simulink model "PropellerModel"  (R2022b)
settings: Solver=VariableStepAuto  StartTime=0.0  StopTime=500  RelTol=1e-3
libraries: mssSimulink x1
settings Model: PacingRate=10  Creator=Lenovo  LastModifiedBy=ADMIN
settings ModelReferenceCC: EnableRefExpFcnMdlSchedulingChecks=on

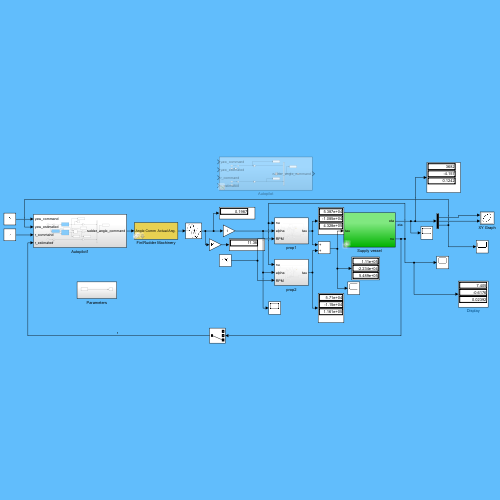
[thumbnail: Simulink's stored preview of the top-level diagram]
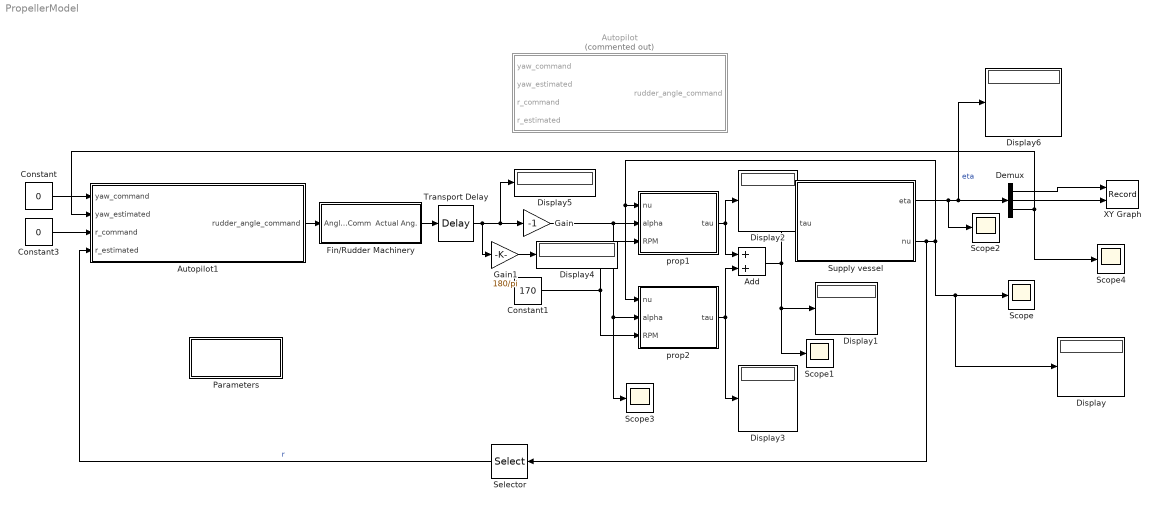
== system PropellerModel ==
  Add : Sum
  Autopilot : Subsystem  Commented=on
  Autopilot1 : Subsystem
  Constant : Constant  Value=0
  Constant1 : Constant  Value=170
  Constant3 : Constant  Value=0
  Demux : Demux  Outputs=3
  Display{,1..6} (7 alike) : Display
  Fin/Rudder Machinery : Subsystem  AncestorBlock=mssSimulink/Modelling/Control Surfaces/Fin//Rudder Machinery  mask(Rudder Machinery){Dmax=20, Dvmax=2*pi*1000/180, tc=.1}
      mask prompts: Dmax "Max. Rudder Angle (rad):"; Dvmax "Max. Rudder Rate (rad/sec.):"; tc "Time constant (sec):"
      mask help:
      | Model of van Amerongen for rudder machiery
      | Copyright (C) 2005 NTNU
      | Author: Tristan Perez
      settings: LibrarySourceBlock=mssSimulink/Modelling/Control Surfaces/Fin//Rudder Machinery
      mask Help: Rudder machinery model of Van Amerongen accounting for saturation and rate limit.
  Gain : Gain  Gain=-1
  Gain1 : Gain  Gain=180/pi
  Parameters : Subsystem
  Scope{,1..4} (5 alike) : Scope
  Selector : Selector  InputPortWidth=3  IndexOptions=Index vector (dialog)  Indices=[3]  OutputSizes=1
  Supply vessel : Subsystem  AncestorBlock=mssSimulink/Marine craft models/Supply vessel
      settings: LibrarySourceBlock=mssSimulink/Marine craft models/Supply vessel
  Transport Delay : TransportDelay  DelayTime=3
  XY Graph : Record  RecordToWorkspace=on  FileSettingsInternal="{\"entries\":[{\"content\":{\"excelSettings\":{\"content\":{},\"type\":\"Streamout.ExcelSettings\"}},\"type\":\"Streamout.FileSettingStorage\",\"uuid\":\"4c8f667d-2ec8-40bb-a75c-241daf6926ec\"}],\"packageUris\":[\"http://schema.mathworks.com/mf0/streamout_blocks/R2020a\"],\"version\":\"1.0\"}"  Layout=[1 1]  SignalsInternal="{\"entries\":[{\"content\":{\"signals\":[{\"content\":{\"blockPath\":[\"PropellerModel/XY Graph\"],\"channel\":[],\"dimensions\":[1],\"domain\":\"PropellerModel/XY Graph\",\"lineColor\":\"#a2142f\",\"plots\":[1],\"port\":1,\"sid\":[\"\"],\"signalID\":30923,\"signalName\":\"Demux:1\"},\"type\":\"RecordBlkView.Signal\",\"uuid\":\"623a59a8-df64-41e8-a8fb-f785ae9d3377\"},{\"content\":{\"blockPath\":[\"PropellerModel/XY Graph\"],\"channel\":[],\"dimensions\":[1],\"domain\":\"PropellerModel/XY Graph\",\"lineColor\":\"#139fff\",\"plots\":[1],\"port\":2,\"sid\":[\"\"],\"signalID\":30927,\"signalName\":\"Demux:2\"},\"type\":\"RecordBlkView.Signal\",\"uuid\":\"a734874c-224f-4494-ab74-00e3b52a102c\"}]},\"type\":\"RecordBlkView.InputSignals\",\"uuid\":\"024bf6ff-c6de-4f18-8bef-f27dde48d678\"}],\"packageUris\":[\"http://schema.mathworks.com/mf0/streamout_blocks/R2020a\"],\"version\":\"1.0\"}"  VisualizationBindings="{\"xyplotplugin\":{\"info\":[{\"series\":[{\"bindingParametersList\":[{\"parameter\":\"X-Axis\",\"signalID\":30923,\"signalName\":\"Demux:1\"},{\"parameter\":\"Y-Axis\",\"signalID\":30927,\"signalName\":\"Demux:2\"}],\"seriesID\":59875}],\"subplotID\":1}]}}"  CompatibilityTag=XY
  prop1 : Subsystem
  prop2 : Subsystem
  wires:
  Supply vessel/2(nu) -> Selector/1, Display/1, Scope/1, prop2/1(nu), prop1/1(nu)
  Autopilot1/1(rudder_angle_command) -> Fin/Rudder Machinery/1(Angle Comm)
  Supply vessel/1(eta) -> Scope2/1, Display6/1, Demux/1  "eta"
  Demux/1 -> XY Graph/1
  Demux/2 -> XY Graph/2
  Constant1/1 -> prop2/3(RPM), prop1/3(RPM)
  prop1/1(tau) -> Add/1, Display2/1
  prop2/1(tau) -> Add/2, Display3/1
  Add/1 -> Scope1/1, Display1/1, Supply vessel/1(tau)
  Fin/Rudder Machinery/1("Actual Ang. ") -> Transport Delay/1
  Constant/1 -> Autopilot1/1(yaw_command)
  Constant3/1 -> Autopilot1/3(r_command)
  Demux/3 -> Scope4/1, Autopilot1/2(yaw_estimated)
  Selector/1 -> Autopilot1/4(r_estimated)  "r"
  Gain/1 -> prop2/2(alpha), Scope3/1, prop1/2(alpha)
  Gain1/1 -> Display4/1
  Transport Delay/1 -> Gain1/1, Display5/1, Gain/1

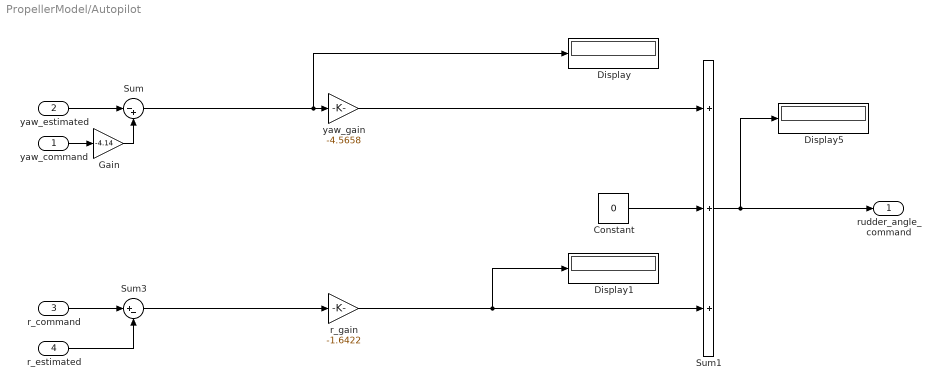
== system PropellerModel/Autopilot ==
  yaw_command : Inport
  yaw_estimated : Inport  Port=2
  r_command : Inport  Port=3
  r_estimated : Inport  Port=4
  Constant : Constant  Value=0
  Display : Display
  Display1 : Display
  Display5 : Display
  Gain : Gain  Gain=-4.14
  Sum : Sum  Inputs=|-+
  Sum1 : Sum  Inputs=+++  InputSameDT=on  SaturateOnIntegerOverflow=on  OutDataTypeStr=Inherit: Same as first input
  Sum3 : Sum  Inputs=|+-  InputSameDT=on  SaturateOnIntegerOverflow=on  OutDataTypeStr=Inherit: Same as first input
  r_gain : Gain  Gain=-1.6422
  yaw_gain : Gain  Gain=-4.5658
  rudder_angle_command : Outport
  wires:
  r_gain/1 -> Display1/1, Sum1/3
  Sum3/1 -> r_gain/1
  Sum1/1 -> Display5/1, rudder_angle_command/1
  r_estimated/1 -> Sum3/2
  r_command/1 -> Sum3/1
  yaw_estimated/1 -> Sum/1
  Sum/1 -> Display/1, yaw_gain/1
  yaw_gain/1 -> Sum1/1
  Constant/1 -> Sum1/2
  yaw_command/1 -> Gain/1
  Gain/1 -> Sum/2

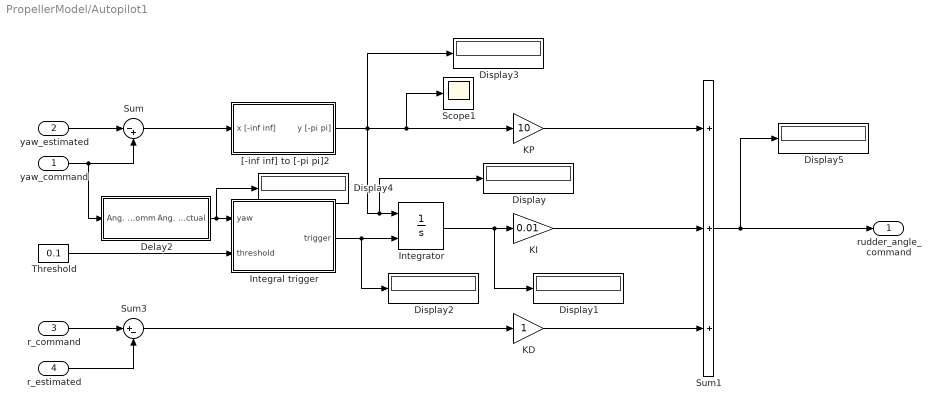
== system PropellerModel/Autopilot1 ==
  yaw_command : Inport
  yaw_estimated : Inport  Port=2
  r_command : Inport  Port=3
  r_estimated : Inport  Port=4
  Delay2 : Subsystem
  Display{,1..5} (6 alike) : Display
  Integral trigger : MATLAB Function  TreatAsAtomicUnit=on
  Integrator : Integrator  ExternalReset=level hold  LimitOutput=on  UpperSaturationLimit=deg2rad(20)  LowerSaturationLimit=deg2rad(-20)
  KD : Gain
  KI : Gain  Gain=0.01
  KP : Gain  Gain=10
  Scope1 : Scope
  Sum : Sum  Inputs=|-+
  Sum1 : Sum  Inputs=+++  InputSameDT=on  SaturateOnIntegerOverflow=on  OutDataTypeStr=Inherit: Same as first input
  Sum3 : Sum  Inputs=|+-  InputSameDT=on  SaturateOnIntegerOverflow=on  OutDataTypeStr=Inherit: Same as first input
  Threshold : Constant  Value=0.1
  "[-inf inf] to [-pi pi]2" : Subsystem  AncestorBlock=mssSimulink/Utilities/Math Operations/[-inf inf] to [-pi pi]  mask([-inf inf] to [-pi pi]){}
      mask help: Converts an angle in rad to (-pi pi)
      settings: LibrarySourceBlock=mssSimulink/Utilities/Math Operations/[-inf inf] to [-pi pi]
  rudder_angle_command : Outport
  wires:
  Integrator/1 -> Display1/1, KI/1
  KD/1 -> Sum1/3
  Sum/1 -> "[-inf inf] to [-pi pi]2"/1(x [-inf inf])
  Sum3/1 -> KD/1
  "[-inf inf] to [-pi pi]2"/1(y [-pi pi]) -> Scope1/1, KP/1, Display3/1, Display/1, Integrator/1
  KI/1 -> Sum1/2
  Sum1/1 -> Display5/1, rudder_angle_command/1
  r_estimated/1 -> Sum3/2
  r_command/1 -> Sum3/1
  yaw_estimated/1 -> Sum/1
  KP/1 -> Sum1/1
  Integral trigger/1(trigger) -> Display2/1, Integrator/2
  Threshold/1 -> Integral trigger/2(threshold)
  yaw_command/1 -> Sum/2, Delay2/1(Ang. Comm)
  Delay2/1(Ang. Actual) -> Display4/1, Integral trigger/1(yaw)

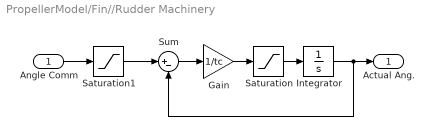
== system PropellerModel/Fin//Rudder Machinery ==
  Angle Comm : Inport
  Gain : Gain  Gain=1/tc  SaturateOnIntegerOverflow=on  OutDataTypeStr=Inherit: Same as input  ParamDataTypeStr=Inherit: Same as input
  Integrator : Integrator
  Saturation : Saturate  UpperLimit=deg2rad(3)  LowerLimit=-deg2rad(3)
  Saturation1 : Saturate  UpperLimit=deg2rad(Dmax)  LowerLimit=deg2rad(-Dmax)
  Sum : Sum  Inputs=|+-  InputSameDT=on  SaturateOnIntegerOverflow=on  OutDataTypeStr=Inherit: Same as first input
  "Actual Ang. " : Outport  VectorParamsAs1DForOutWhenUnconnected=off
  wires:
  Gain/1 -> Saturation/1
  Sum/1 -> Gain/1
  Integrator/1 -> Sum/2, "Actual Ang. "/1
  Saturation1/1 -> Sum/1
  Saturation/1 -> Integrator/1
  Angle Comm/1 -> Saturation1/1

== system PropellerModel/Parameters ==
  Mass : Constant  Value=357.0*1014
  tag scope: Mass=global
  wires:
  Mass/1 -> [Mass]

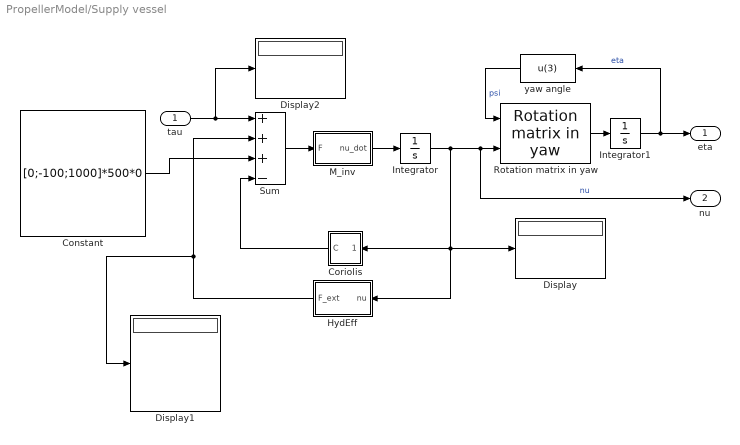
== system PropellerModel/Supply vessel ==
  tau : Inport
  Constant : Constant  Value=[0;-100;1000]*500*0
  Coriolis : Subsystem
  Display : Display
  Display1 : Display
  Display2 : Display
  HydEff : Subsystem
  Integrator : Integrator  InitialCondition=[0 1 0]
  Integrator1 : Integrator
  M_inv : Subsystem
  "Rotation matrix in yaw " : mssSimulink/Modelling/Kinematics/Rotation matrix in yaw 
  Sum : Sum  Inputs=+++-  InputSameDT=on  SaturateOnIntegerOverflow=on  OutDataTypeStr=Inherit: Same as first input
  yaw angle : Fcn  Expr=u(3)
  eta : Outport  InitialOutput=0  VectorParamsAs1DForOutWhenUnconnected=off
  nu : Outport  Port=2  InitialOutput=0  VectorParamsAs1DForOutWhenUnconnected=off
  wires:
  Sum/1 -> M_inv/1(F)
  M_inv/1(nu_dot) -> Integrator/1
  tau/1 -> Display2/1, Sum/1
  "Rotation matrix in yaw "/1 -> Integrator1/1
  yaw angle/1 -> "Rotation matrix in yaw "/1  "psi"
  Integrator/1 -> Display/1, HydEff/1(nu), Coriolis/1(nu), "Rotation matrix in yaw "/2, nu/1  "nu"
  Integrator1/1 -> yaw angle/1, eta/1  "eta"
  HydEff/1(F_ext) -> Display1/1, Sum/2
  Coriolis/1(C) -> Sum/4
  Constant/1 -> Sum/3

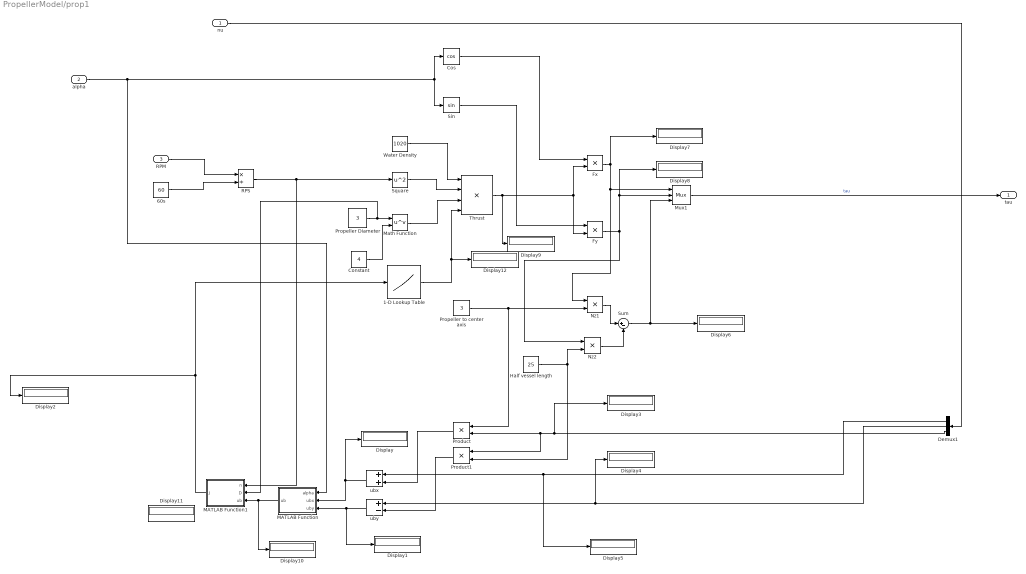
== system PropellerModel/prop1 ==
  nu : Inport
  alpha : Inport  Port=2
  RPM : Inport  Port=3
  1-D Lookup Table : Lookup_n-D  NumberOfTableDimensions=1  BreakpointsForDimension1=[0:0.05:1.05]  Table=-0.3*[0:0.05:1.05]+0.35  InternalRulePriority=Speed  RndMeth=Simplest
  60s : Constant  Value=60
  Constant : Constant  Value=4
  Cos : Trigonometry  Operator=cos
  Demux1 : Demux  Outputs=3
  Display{,1..12} (13 alike) : Display
  Fx : Product
  Fy : Product
  Half vessel length : Constant  Value=25
  MATLAB Function : MATLAB Function  TreatAsAtomicUnit=on
  MATLAB Function1 : MATLAB Function  TreatAsAtomicUnit=on
  Math Function : Math  Operator=pow
  Mux1 : Mux  Inputs=3
  Nz1 : Product
  Nz2 : Product
  Product : Product
  Product1 : Product
  "Propeller Diameter " : Constant  Value=3
  Propeller to center axis : Constant  Value=3
  RPS : Product  Inputs=*/  RndMeth=Zero  SaturateOnIntegerOverflow=on
  Sin : Trigonometry
  Square : Math  Operator=square
  Sum : Sum  Inputs=|+-
  Thrust : Product  Inputs=4
  Water Density : Constant  Value=1020
  ubx : Sum
  uby : Sum  Inputs=+-
  tau : Outport
  wires:
  nu/1 -> Demux1/1
  Nz2/1 -> Sum/2
  alpha/1 -> Cos/1, Sin/1, MATLAB Function/1(alpha)
  RPS/1 -> Square/1, MATLAB Function1/1(n)
  Half vessel length/1 -> Product1/2, Nz2/2
  Fy/1 -> Display8/1, Mux1/2, Nz2/1
  Water Density/1 -> Thrust/1
  uby/1 -> MATLAB Function/3(uby), Display1/1
  Propeller to center axis/1 -> Product/1, Nz1/2
  Thrust/1 -> Display9/1, Fy/2, Fx/2
  Fx/1 -> Mux1/1, Nz1/1, Display7/1
  Square/1 -> Thrust/2
  Demux1/2 -> Display4/1, uby/1
  MATLAB Function/1(ub) -> Display10/1, MATLAB Function1/3(ub)
  60s/1 -> RPS/2
  Cos/1 -> Fx/1
  Demux1/1 -> Display5/1, ubx/1
  Sum/1 -> Display6/1, Mux1/3
  ubx/1 -> MATLAB Function/2(ubx), Display/1
  Nz1/1 -> Sum/1
  MATLAB Function1/1(J) -> 1-D Lookup Table/1, Display2/1
  1-D Lookup Table/1 -> Thrust/4, Display12/1
  Mux1/1 -> tau/1  "tau"
  RPM/1 -> RPS/1
  Demux1/3 -> Display3/1, Product1/1, Product/2
  Product/1 -> ubx/2
  Product1/1 -> uby/2
  Sin/1 -> Fy/1
  "Propeller Diameter "/1 -> Math Function/1, MATLAB Function1/2(D)
  Constant/1 -> Math Function/2
  Math Function/1 -> Thrust/3

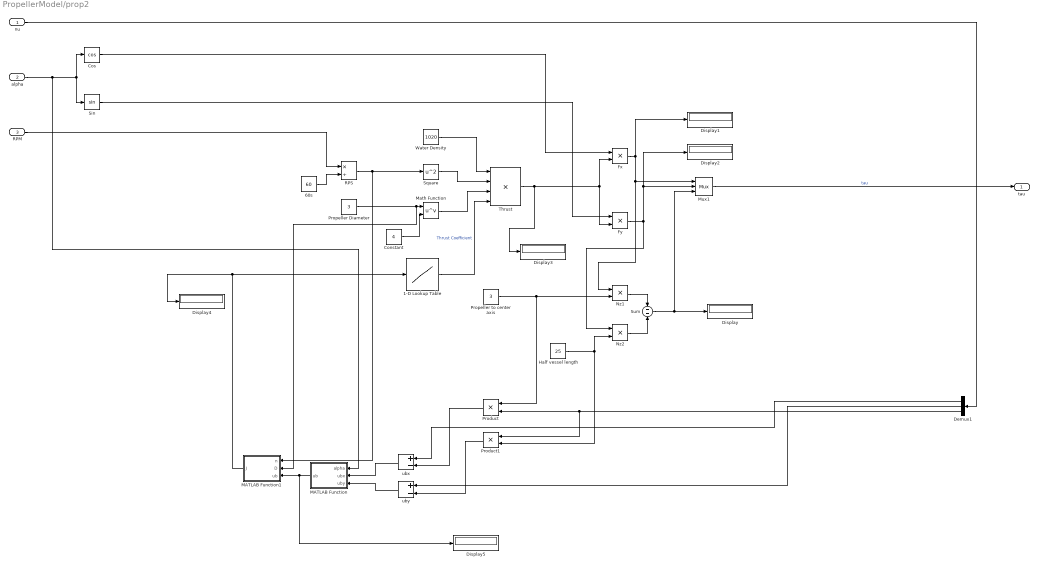
== system PropellerModel/prop2 ==
  nu : Inport
  alpha : Inport  Port=2
  RPM : Inport  Port=3
  1-D Lookup Table : Lookup_n-D  NumberOfTableDimensions=1  BreakpointsForDimension1=[0:0.05:1.05]  Table=-0.3*[0:0.05:1.05]+0.35  InternalRulePriority=Speed  RndMeth=Simplest
  60s : Constant  Value=60
  Constant : Constant  Value=4
  Cos : Trigonometry  Operator=cos
  Demux1 : Demux  Outputs=3
  Display{,1..5} (6 alike) : Display
  Fx : Product
  Fy : Product
  Half vessel length : Constant  Value=25
  MATLAB Function : MATLAB Function  TreatAsAtomicUnit=on
  MATLAB Function1 : MATLAB Function  TreatAsAtomicUnit=on
  Math Function : Math  Operator=pow
  Mux1 : Mux  Inputs=3
  Nz1 : Product
  Nz2 : Product
  Product : Product
  Product1 : Product
  Propeller Diameter : Constant  Value=3
  Propeller to center axis : Constant  Value=3
  RPS : Product  Inputs=*/  RndMeth=Zero  SaturateOnIntegerOverflow=on
  Sin : Trigonometry
  Square : Math  Operator=square
  Sum : Sum  Inputs=--
  Thrust : Product  Inputs=4
  Water Density : Constant  Value=1020
  ubx : Sum  Inputs=+-
  uby : Sum  Inputs=+-
  tau : Outport
  wires:
  Product1/1 -> uby/2
  Product/1 -> ubx/2
  Demux1/3 -> Product1/1, Product/2
  RPM/1 -> RPS/1
  Mux1/1 -> tau/1  "tau"
  1-D Lookup Table/1 -> Thrust/4  "Thrust Coefficient"
  MATLAB Function1/1(J) -> Display4/1, 1-D Lookup Table/1
  Nz1/1 -> Sum/1
  Sum/1 -> Mux1/3, Display/1
  60s/1 -> RPS/2
  Demux1/2 -> uby/1
  Square/1 -> Thrust/2
  Propeller Diameter/1 -> MATLAB Function1/2(D), Math Function/1
  Fx/1 -> Nz1/1, Mux1/1, Display1/1
  Thrust/1 -> Display3/1, Fx/2, Fy/2
  Propeller to center axis/1 -> Nz1/2, Product/1
  Water Density/1 -> Thrust/1
  Fy/1 -> Nz2/1, Display2/1, Mux1/2
  Half vessel length/1 -> Nz2/2, Product1/2
  RPS/1 -> Square/1, MATLAB Function1/1(n)
  alpha/1 -> MATLAB Function/1(alpha), Sin/1, Cos/1
  Nz2/1 -> Sum/2
  nu/1 -> Demux1/1
  Cos/1 -> Fx/1
  Sin/1 -> Fy/1
  Math Function/1 -> Thrust/3
  Constant/1 -> Math Function/2
  Demux1/1 -> ubx/1
  ubx/1 -> MATLAB Function/2(ubx)
  uby/1 -> MATLAB Function/3(uby)
  MATLAB Function/1(ub) -> Display5/1, MATLAB Function1/3(ub)

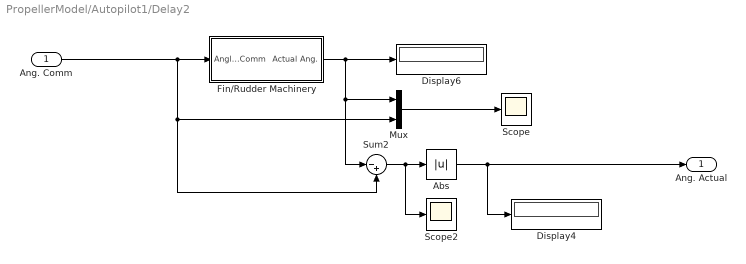
== system PropellerModel/Autopilot1/Delay2 ==
  Ang. Comm : Inport
  Abs : Abs  SaturateOnIntegerOverflow=off
  Display4 : Display
  Display6 : Display
  Fin/Rudder Machinery : Subsystem  AncestorBlock=mssSimulink/Modelling/Control Surfaces/Fin//Rudder Machinery  mask(Rudder Machinery){Dmax=20, Dvmax=0.05, tc=.005}
      mask prompts: Dmax "Max. Rudder Angle (rad):"; Dvmax "Max. Rudder Rate (rad/sec.):"; tc "Time constant (sec):"
      mask help:
      | Model of van Amerongen for rudder machiery
      | Copyright (C) 2005 NTNU
      | Author: Tristan Perez
      settings: LibrarySourceBlock=mssSimulink/Modelling/Control Surfaces/Fin//Rudder Machinery
      mask Help: Rudder machinery model of Van Amerongen accounting for saturation and rate limit.
  Mux : Mux  Inputs=2
  Scope : Scope
  Scope2 : Scope
  Sum2 : Sum  Inputs=|-+
  Ang. Actual : Outport
  wires:
  Sum2/1 -> Scope2/1, Abs/1
  Ang. Comm/1 -> Fin/Rudder Machinery/1(Angle Comm), Sum2/2, Mux/2
  Fin/Rudder Machinery/1("Actual Ang. ") -> Sum2/1, Mux/1, Display6/1
  Abs/1 -> Ang. Actual/1, Display4/1
  Mux/1 -> Scope/1

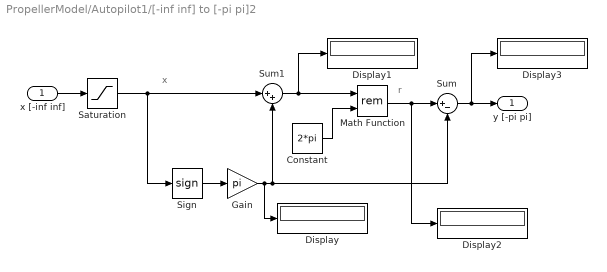
== system PropellerModel/Autopilot1/[-inf inf] to [-pi pi]2 ==
  note: x
  note: r
  x [-inf inf] : Inport
  Constant : Constant  Value=2*pi
  Display{,1..3} (4 alike) : Display
  Gain : Gain  Gain=pi  SaturateOnIntegerOverflow=on  OutDataTypeStr=Inherit: Same as input  ParamDataTypeStr=Inherit: Same as input
  Math Function : Math  Operator=rem  SignedPower=on
  Saturation : Saturate  UpperLimit=1e10  LowerLimit=-1e10
  Sign : Signum
  Sum : Sum  Inputs=|+-  SaturateOnIntegerOverflow=on
  Sum1 : Sum  Inputs=|++  SaturateOnIntegerOverflow=on
  y [-pi pi] : Outport  VectorParamsAs1DForOutWhenUnconnected=off
  wires:
  x [-inf inf]/1 -> Saturation/1
  Sign/1 -> Gain/1
  Gain/1 -> Display/1, Sum/2, Sum1/2
  Sum1/1 -> Display1/1, Math Function/1
  Constant/1 -> Math Function/2
  Sum/1 -> Display3/1, y [-pi pi]/1
  Saturation/1 -> Sum1/1, Sign/1
  Math Function/1 -> Display2/1, Sum/1

== system PropellerModel/Supply vessel/Coriolis ==
  nu : Inport
  Demux : Demux  Outputs=3
  Display : Display
  MATLAB Function : MATLAB Function  TreatAsAtomicUnit=on
  Mux : Mux  Inputs=3
  C : Outport
  wires:
  nu/1 -> Display/1, Demux/1
  MATLAB Function/2(C2) -> Mux/2
  MATLAB Function/3(C3) -> Mux/3
  MATLAB Function/1(C1) -> Mux/1
  Mux/1 -> C/1
  Demux/1 -> MATLAB Function/1(u)
  Demux/2 -> MATLAB Function/2(v)
  Demux/3 -> MATLAB Function/3(r)

== system PropellerModel/Supply vessel/HydEff ==
  nu : Inport
  Bus Creator : BusCreator  Inputs=3
  Demux : Demux  Outputs=3
  MATLAB Function : MATLAB Function  TreatAsAtomicUnit=on
  F_ext : Outport
  wires:
  [Mass] -> MATLAB Function/1(mass)
  MATLAB Function/1(Xh) -> Bus Creator/1
  Bus Creator/1 -> F_ext/1
  MATLAB Function/2(Yh) -> Bus Creator/2
  MATLAB Function/3(Nh) -> Bus Creator/3
  nu/1 -> Demux/1
  Demux/1 -> MATLAB Function/2(u)
  Demux/2 -> MATLAB Function/3(v)
  Demux/3 -> MATLAB Function/4(r)

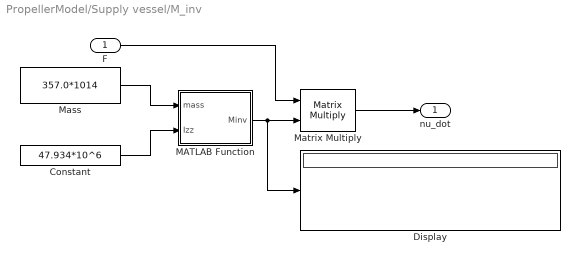
== system PropellerModel/Supply vessel/M_inv ==
  F : Inport
  Constant : Constant  Value=47.934*10^6
  Display : Display
  MATLAB Function : MATLAB Function  TreatAsAtomicUnit=on
  Mass : Constant  Value=357.0*1014
  Matrix Multiply : Product  Multiplication=Matrix(*)
  nu_dot : Outport
  wires:
  MATLAB Function/1(Minv) -> Display/1, Matrix Multiply/2
  Mass/1 -> MATLAB Function/1(mass)
  Constant/1 -> MATLAB Function/2(Izz)
  Matrix Multiply/1 -> nu_dot/1
  F/1 -> Matrix Multiply/1

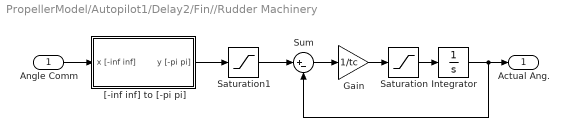
== system PropellerModel/Autopilot1/Delay2/Fin//Rudder Machinery ==
  Angle Comm : Inport
  Gain : Gain  Gain=1/tc  SaturateOnIntegerOverflow=on  OutDataTypeStr=Inherit: Same as input  ParamDataTypeStr=Inherit: Same as input
  Integrator : Integrator
  Saturation : Saturate  UpperLimit=Dvmax  LowerLimit=-Dvmax
  Saturation1 : Saturate  UpperLimit=Dmax  LowerLimit=-Dmax
  Sum : Sum  Inputs=|+-  InputSameDT=on  SaturateOnIntegerOverflow=on  OutDataTypeStr=Inherit: Same as first input
  "[-inf inf] to [-pi pi]" : Subsystem  AncestorBlock=mssSimulink/Utilities/Math Operations/[-inf inf] to [-pi pi]  mask([-inf inf] to [-pi pi]){}
      mask help: Converts an angle in rad to (-pi pi)
      settings: LibrarySourceBlock=mssSimulink/Utilities/Math Operations/[-inf inf] to [-pi pi]
  "Actual Ang. " : Outport  VectorParamsAs1DForOutWhenUnconnected=off
  wires:
  Gain/1 -> Saturation/1
  Sum/1 -> Gain/1
  Integrator/1 -> Sum/2, "Actual Ang. "/1
  Saturation1/1 -> Sum/1
  Saturation/1 -> Integrator/1
  Angle Comm/1 -> "[-inf inf] to [-pi pi]"/1(x [-inf inf])
  "[-inf inf] to [-pi pi]"/1(y [-pi pi]) -> Saturation1/1

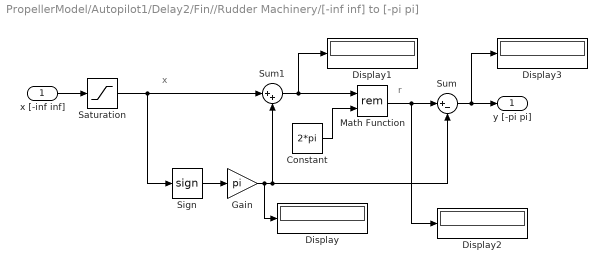
== system PropellerModel/Autopilot1/Delay2/Fin//Rudder Machinery/[-inf inf] to [-pi pi] ==
  note: x
  note: r
  x [-inf inf] : Inport
  Constant : Constant  Value=2*pi
  Display{,1..3} (4 alike) : Display
  Gain : Gain  Gain=pi  SaturateOnIntegerOverflow=on  OutDataTypeStr=Inherit: Same as input  ParamDataTypeStr=Inherit: Same as input
  Math Function : Math  Operator=rem  SignedPower=on
  Saturation : Saturate  UpperLimit=1e10  LowerLimit=-1e10
  Sign : Signum
  Sum : Sum  Inputs=|+-  SaturateOnIntegerOverflow=on
  Sum1 : Sum  Inputs=|++  SaturateOnIntegerOverflow=on
  y [-pi pi] : Outport  VectorParamsAs1DForOutWhenUnconnected=off
  wires:
  x [-inf inf]/1 -> Saturation/1
  Sign/1 -> Gain/1
  Gain/1 -> Display/1, Sum/2, Sum1/2
  Sum1/1 -> Display1/1, Math Function/1
  Constant/1 -> Math Function/2
  Sum/1 -> Display3/1, y [-pi pi]/1
  Saturation/1 -> Sum1/1, Sign/1
  Math Function/1 -> Display2/1, Sum/1

== matlab function PropellerModel/Supply vessel/Coriolis/MATLAB Function ==
  data: u input; C1 output; C2 output; C3 output; v input; r input
function [C1,    C2,    C3]    = fcn(u,v,r)

% u = nu(1);
% v = nu(2);
% r = nu(3);

x_g = 0;
m = 357.0*1014;

C = [0                 0  -m*(x_g*r + v); ...
     0                 0             m*u; ...
     m*(x_g*r + v)  -m*u              0];

Co = C*[u;v;r];
C1 = Co(1);
C2 = Co(2);
C3 = Co(3);

end

% Xc =   h.m*(r*v+h.xG*r^2-h.zG*p*r);  
% Yc = - h.m*u*r;
% Kc =   h.m*h.zG*u*r;
% Nc = - h.m*h.xG*u*r;

== matlab function PropellerModel/prop1/MATLAB Function ==
  data: alpha input; ubx input; ub output; uby input
function ub = fcn(alpha, ubx, uby)
    
    phi = atan(uby/ubx);
    beta = phi - alpha;
    ub = abs(hypot(ubx,uby)*cos(beta));

end

== matlab function PropellerModel/Supply vessel/M_inv/MATLAB Function ==
  data: Minv output; mass input; Izz input
function Minv = fcn(mass, Izz)

h.m   = mass;    % Mass [Kg]
h.Izz = Izz;     % Yaw Inertia
h.xG  = 0;

%%%%%%%%%%%%%%%%%%%%%%%%%%%%%%%%%%%%%%%%%%%%%%%%%%%%%%%%%%%%%%%%%%%%%%%
% The hydrodynamic derivatives are given in dimensional form, and follow
% from the original publication of Blanke and Christensen 1993.
%%%%%%%%%%%%%%%%%%%%%%%%%%%%%%%%%%%%%%%%%%%%%%%%%%%%%%%%%%%%%%%%%%%%%%%
% Data for surge equation 
h.Xudot  	= -17400.0;
% h.Xuau     	= -1.96e+003;
% h.Xvr    	=  0.33 * mass;
   
% Hydrodynamic coefficients in sway equation
h.Yvdot = -393000; 
h.Ypdot = -296000; 
h.Yrdot = -1400000; 
% h.Yauv  = -11800; 
% h.Yur   =  131000; 
% h.Yvav  = -3700; 
% h.Yrar  =  0;
% h.Yvar  = -794000; 
% h.Yrav  = -182000; 
% h.Ybauv =  10800; % Y_{\phi |v u|}
% h.Ybaur =  251000; 
% h.Ybuu  = -74;


% Hydrodynamic coefficients in yaw equation
h.Nvdot =  538000;
h.Npdot =  0;
h.Nrdot = -38.7e6;
% h.Nauv  = -92000;
% h.Naur  = -4710000;
% h.Nvav  =  0;
% h.Nrar  = -202000000;
% h.Nvar  =  0;
% h.Nrav  = -15600000;
% h.Nbauv = -214000;
% h.Nbuar = -4980000;
% h.Nbuau = -8000;
%%%%%%%%%%%%%%%%%%%%%%%%%%%%%%%%%%%%%%%%%%%%%%%%%%%%%%%%%%%%%%%%%%%%%%%%%%%


M = [(h.m-h.Xudot)                  0                  0; ...
                 0      (h.m-h.Yvdot) (h.m*h.xG-h.Yrdot); ...
                 0 (h.m*h.xG-h.Nvdot)    (h.Izz-h.Nrdot)];

Minv = inv(M);
end

== matlab function PropellerModel/Supply vessel/HydEff/MATLAB Function ==
  data: mass input; Xh output; Yh output; Nh output; u input; v input; r input
function [Xh, Yh, Nh] = fcn(mass, u, v, r)

%%%%%%%%%%%%%%%%%%%%%%%%%%%%%%%%%%%%%%%%%%%%%%%%%%%%%%%%%%%%%%%%%%%%%%%
% The hydrodynamic derivatives are given in dimensional form, and follow
% from the original publication of Blanke and Christensen 1993.
%%%%%%%%%%%%%%%%%%%%%%%%%%%%%%%%%%%%%%%%%%%%%%%%%%%%%%%%%%%%%%%%%%%%%%%
% Data for surge equation 
h.Xudot  	= -17400.0 ;
h.Xuau     	= -1.96e+003 ;
h.Xvr    	=  0.33 * mass ;
   
% Hydrodynamic coefficients in sway equation
h.Yvdot = -393000 ; 
h.Ypdot = -296000 ; 
h.Yrdot = -1400000 ; 
h.Yauv  = -11800 ; 
h.Yur   =  131000 ; 
h.Yvav  = -3700 ; 
h.Yrar   =  0 ;
h.Yvar  = -794000 ; 
h.Yrav  = -182000 ; 
h.Ybauv =  10800 ; % Y_{\phi |v u|}
h.Ybaur =  251000 ; 
h.Ybuu  = -74 ; 


% Hydrodynamic coefficients in yaw equation
h.Nvdot =  538000 ;
h.Npdot =  0 ;
h.Nrdot = -38.7e6;
h.Nauv  = -92000 ;
h.Naur  = -4710000 ;
h.Nvav  =  0 ;
h.Nrar  = -202000000 ;
h.Nvar  =  0 ;
h.Nrav  = -15600000 ;
h.Nbauv = -214000 ;
h.Nbuar = -4980000 ;
h.Nbuau = -8000 ;
%%%%%%%%%%%%%%%%%%%%%%%%%%%%%%%%%%%%%%%%%%%%%%%%%%%%%%%%%%%%%%%%%%%%%%%%%%%

au = abs(u);
av = abs(v); 
ar = abs(r);
b = 0;

% Hydrodynamic forces without added mass terms (considered in the M matrix)
Xh  = h.Xuau*u*au+h.Xvr*v*r;

Yh = h.Yauv*au*v + h.Yur*u*r + h.Yvav*v*av + h.Yvar*v*ar + h.Yrav*r*av ...
   + h.Ybauv*b*abs(u*v) + h.Ybaur*b*abs(u*r) + h.Ybuu*b*u^2;

Nh = h.Nauv*au*v + h.Naur*au*r + h.Nrar*r*ar + h.Nrav*r*av...
   +h.Nbauv*b*abs(u*b) + h.Nbuar*b*u*ar + h.Nbuau*b*u*au;

end

== matlab function PropellerModel/prop1/MATLAB Function1 ==
  data: n input; D input; ub input; J output
function J = fcn(n,D,ub)
    J =ub/(n*D) ;
end

== matlab function PropellerModel/prop2/MATLAB Function ==
  data: alpha input; ubx input; ub output; uby input
function ub = fcn(alpha, ubx, uby)
    
    phi = atan(uby/ubx);
    beta = phi - alpha;
    ub = abs(hypot(ubx,uby)*cos(beta));

end

== matlab function PropellerModel/prop2/MATLAB Function1 ==
  data: n input; D input; ub input; J output
function J = fcn(n,D,ub)
    J =ub/(n*D) ;
end

== matlab function PropellerModel/Autopilot1/Integral trigger ==
  data: yaw input; trigger output; threshold input
function trigger = fcn(yaw, threshold)

if abs(yaw) < threshold
   trigger = 0;   % Trigger Integral part of PID
else
   trigger = 1;   % Stop Integral part of PID
end

end
